simulink subsystem "TOAD_TrajectoryGen_3"  (R2026a)
settings: Solver=VariableStepAuto
values from neighbouring files (symbols this model uses):
  constants6DoF = LoadTOADParams(Vehicle)    [TrajectoryGenerator.m]    (also in TrajectoryGeneratorHybrid.m)
settings Model: Creator=pplat  LastModifiedBy=pplat

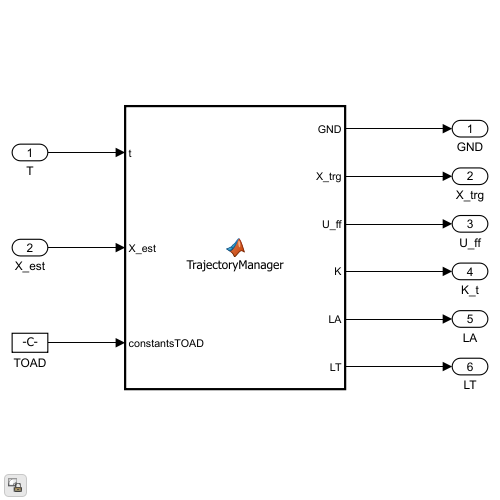
[thumbnail: Simulink's stored preview of the top-level diagram]
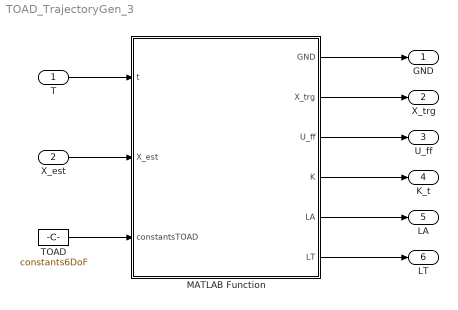
== system TOAD_TrajectoryGen_3 ==
  T : Inport
  X_est : Inport  Port=2
  MATLAB Function : MATLAB Function  TreatAsAtomicUnit=on
  TOAD : Constant  Value=constants6DoF  OutDataTypeStr=Bus: Vehicle_Bus
  GND : Outport
  X_trg : Outport  Port=2
  U_ff : Outport  Port=3
  K_t : Outport  Port=4
  LA : Outport  Port=5
  LT : Outport  Port=6
  wires:
  T/1 -> MATLAB Function/1(t)
  MATLAB Function/2(X_trg) -> X_trg/1
  MATLAB Function/3(U_ff) -> U_ff/1
  MATLAB Function/4(K) -> K_t/1
  MATLAB Function/1(GND) -> GND/1
  MATLAB Function/6(LT) -> LT/1
  MATLAB Function/5(LA) -> LA/1
  TOAD/1 -> MATLAB Function/3(constantsTOAD)
  X_est/1 -> MATLAB Function/2(X_est)

== matlab function TOAD_TrajectoryGen_3/MATLAB Function ==
  data: GND output; t input; X_trg output; U_ff output; K output; X_est input; LA output; LT output; constantsTOAD input
function [GND, X_trg, U_ff, K, LA, LT] = TrajectoryManager(t, X_est, constantsTOAD)
    
    %% GND mode handling 
    PadHoldTime = 10;
    MET = t - PadHoldTime;
    GND = 1;
    if MET < 0
        MET = 0;
    else
        GND = 0;
    end

    % Call the trajectory manager
    [X_trg, U_ff, K, LA, LT] = TrajectoryManager(MET, X_est, constantsTOAD);
end
